simulink model "Sim_Induct_Harmon"  (R2019a)
settings: Solver=FixedStepAuto  StartTime=0.0  StopTime=sim_time  FixedStep=1e-6  MaxStep=1e-4  RelTol=1e-3
values from neighbouring files (symbols this model uses):
  J = 0.0025    [motor_parameters.mat]
  Laq = 0.001    [motor_parameters.mat]
  Lse = 0.001    [motor_parameters.mat]
  Ra = 2.08    [motor_parameters.mat]
  Rse = 5.7    [motor_parameters.mat]
  SEIP4 = [-14.225 -12.275 -10.725 -9.725 -9.1 -8.6 -8.075 -7.65 -7.2 -6.85 -6.492 -6.135 ... (45 elements, 1x45)]    [motor_parameters.mat]
  SEVP4 = [-160 -155 -150 -145 -140 -135 -130 -125 -120 -115 -110 -105 ... (45 elements, 1x45)]    [motor_parameters.mat]
  sim_off = sim_on    [double_load.m]    (also in fourfold_load.m; individual_load.m; triple_load.m)
  sim_on = 50*ones(1,28)    [double_load.m]    (also in fourfold_load.m; individual_load.m; triple_load.m)
  wm0 = 0    [motor_parameters.mat]
  wmo = 157.079632679    [motor_parameters.mat]
undefined symbols (not defined in the file or in its folder): C21, C22, C23, C24, L41, L42, L43, L44, L61, L62, L63, L64, R, R21, R22, R23, R24, R31, R32, R33, R34, R41, R42, R43, R44, R51, R52, R53, R54, R61, R62, R63, R64, R71, R72, R73, R74, Valpha5, Valpha6
libraries: powerlib x225, simulink x72
(part 1 of 3)
settings Model: Creator=USUARIO  LastModifiedBy=USUARIO
settings SolverCC: DecoupledContinuousIntegration=on
settings DataIOCC: ReturnWorkspaceOutputs=off
settings DebuggingCC: ArithmeticOperatorsInVariantConditions=warning
settings SFSimCC: SimUseLocalCustomCode=off
settings RTWCC: RTWUseLocalCustomCode=off

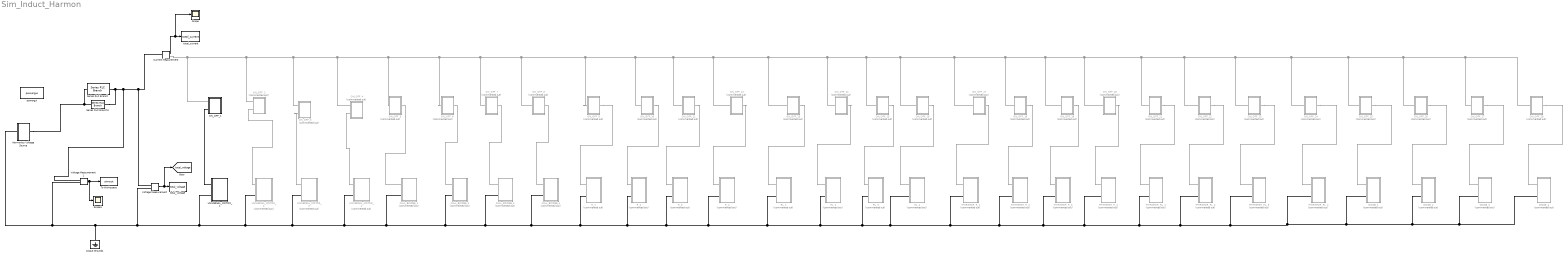
== system Sim_Induct_Harmon ==
  Current Measurement : powerlib/Measurements/Current Measurement  PhasorSimulation=off  OutputType=Complex  PSBequivalent=0
      settings: SourceProductName=Simscape Electrical
  DIODE_1 : Subsystem  Commented=on
  DIODE_2 : Subsystem  Commented=on
  DIODE_3 : Subsystem  Commented=on
  DIODE_4 : Subsystem  Commented=on
  FULL_BRIDGE_1 : Subsystem  Commented=on
  FULL_BRIDGE_2 : Subsystem  Commented=on
  FULL_BRIDGE_3 : Subsystem  Commented=on
  FULL_BRIDGE_4 : Subsystem  Commented=on
  Harmonics Voltage Source : Subsystem
  ON_OFF_1 : Subsystem
  ON_OFF_10 : Subsystem  Commented=on
  ON_OFF_11 : Subsystem  Commented=on
  ON_OFF_12 : Subsystem  Commented=on
  ON_OFF_13 : Subsystem  Commented=on
  ON_OFF_14 : Subsystem  Commented=on
  ON_OFF_15 : Subsystem  Commented=on
  ON_OFF_16 : Subsystem  Commented=on
  ON_OFF_17 : Subsystem  Commented=on
  ON_OFF_18 : Subsystem  Commented=on
  ON_OFF_19 : Subsystem  Commented=on
  ON_OFF_2 : Subsystem  Commented=on
  ON_OFF_20 : Subsystem  Commented=on
  ON_OFF_21 : Subsystem  Commented=on
  ON_OFF_22 : Subsystem  Commented=on
  ON_OFF_23 : Subsystem  Commented=on
  ON_OFF_24 : Subsystem  Commented=on
  ON_OFF_25 : Subsystem  Commented=on
  ON_OFF_26 : Subsystem  Commented=on
  ON_OFF_27 : Subsystem  Commented=on
  ON_OFF_28 : Subsystem  Commented=on
  ON_OFF_3 : Subsystem  Commented=on
  ON_OFF_4 : Subsystem  Commented=on
  ON_OFF_5 : Subsystem  Commented=on
  ON_OFF_6 : Subsystem  Commented=on
  ON_OFF_7 : Subsystem  Commented=on
  ON_OFF_8 : Subsystem  Commented=on
  ON_OFF_9 : Subsystem  Commented=on
  RL_1 : Subsystem  Commented=on
  RL_2 : Subsystem  Commented=on
  RL_3 : Subsystem  Commented=on
  RL_4 : Subsystem  Commented=on
  R_1 : Subsystem  Commented=on
  R_2 : Subsystem  Commented=on
  R_3 : Subsystem  Commented=on
  R_4 : Subsystem  Commented=on
  Scope : Scope
  Scope1 : Scope
  Series RLC Branch : powerlib/Elements/Series RLC Branch  LConnTagsString=__new0  RConnTagsString=__new0  BranchType=RL  Resistance=1e-3  Inductance=1e-3  SetiL0=off  InitialCurrent=0  Capacitance=1e-6  Setx0=off  InitialVoltage=0  Measurements=None
      settings: SourceProductName=Simscape Electrical
  Series RLC Branch1 : powerlib/Elements/Series RLC Branch  LConnTagsString=__new0  RConnTagsString=__new0  BranchType=R  Resistance=3.75e-7  Inductance=1e-12  SetiL0=off  InitialCurrent=0  Capacitance=1e-6  Setx0=off  InitialVoltage=0  Measurements=None
      settings: SourceProductName=Simscape Electrical
  THYRISTOR_RL_1 : Subsystem  Commented=on
  THYRISTOR_RL_2 : Subsystem  Commented=on
  THYRISTOR_RL_3 : Subsystem  Commented=on
  THYRISTOR_RL_4 : Subsystem  Commented=on
  THYRISTOR_R_1 : Subsystem  Commented=on
  THYRISTOR_R_2 : Subsystem  Commented=on
  THYRISTOR_R_3 : Subsystem  Commented=on
  THYRISTOR_R_4 : Subsystem  Commented=on
  To Workspace : ToWorkspace  VariableName=simout  SampleTime=-1
  UNIVERSAL_MOTOR_1 : Subsystem
  UNIVERSAL_MOTOR_2 : Subsystem  Commented=on
  UNIVERSAL_MOTOR_3 : Subsystem  Commented=on
  UNIVERSAL_MOTOR_4 : Subsystem  Commented=on
  Voltage Measurement : powerlib/Measurements/Voltage Measurement  PhasorSimulation=off  OutputType=Complex  PSBequivalent=0
      settings: SourceProductName=Simscape Electrical
  Voltage Measurement1 : powerlib/Measurements/Voltage Measurement  PhasorSimulation=off  OutputType=Complex  PSBequivalent=0
      settings: SourceProductName=Simscape Electrical
  output Ground1 : powerlib/Elements/Ground  LConnTagsString=a
      settings: SourceProductName=Simscape Electrical
  powergui : powerlib/powergui  Priority=1  SimulationMode=Discrete  SampleTime=1e-6  frequency=60  Iterations=100  frequencyindice=0  Pbase=100e6  ErrMax=1e-4  UnitsV=kV  UnitsW=MW  buscounter=0  FunctionMessages=off  echomessages=off  EnableUseOfTLC=off  CurrentSourceSwitches=off  DisableSnubberDevices=off  DisableRonSwitches=off  DisableVfSwitches=off  DisplayEquations=off  AutomaticDiscreteSolvers=off  SolverType=Tustin/Backward Euler (TBE)  Interpol=off  ExternalGateDelay=off  methode=off  Ts=100  x0status=blocks  SPID=off  SwTol=0  HookPort=off  NonlinearTolerance=0  nMaxIteration=15  ContinueOnMaxIteration=off  RestoreLinks=warning  ResistiveCurrentMeasurement=off  Frange=[0:2:500]  Ylog=off  Xlog=on  ShowGrid=off  save=off  variable=ZData  structure=0  ZoomFFT=off  StartTime=0.0  cycles=1  DisplayStyle=1  fundamental=60  FreqAxis=off  MaxFrequency=1000  frequencyindicesteady=1  RmsSteady=1  display=off
      settings: SourceProductName=Simscape Electrical
  total_current : ToWorkspace  VariableName=total_current  SampleTime=-1
  total_voltage : ToWorkspace  VariableName=total_voltage  SampleTime=-1
  tag scope: total_voltage=global
  wires:
  Current Measurement/1 -> Scope/1, total_current/1
  Voltage Measurement/1 -> [total_voltage], total_voltage/1
  Voltage Measurement1/1 -> Scope1/1, To Workspace/1
  connections:
  Harmonics Voltage Source/LConn1 -- Voltage Measurement1/LConn2 -- output Ground1/LConn1 -- Voltage Measurement/LConn2 -- UNIVERSAL_MOTOR_1/LConn2 -- UNIVERSAL_MOTOR_2/LConn2 -- UNIVERSAL_MOTOR_3/LConn2 -- UNIVERSAL_MOTOR_4/LConn2 -- FULL_BRIDGE_4/LConn2 -- R_1/LConn2 -- R_4/LConn2 -- RL_4/LConn2 -- THYRISTOR_R_2/LConn2 -- THYRISTOR_RL_2/LConn2 -- DIODE_3/LConn2 -- DIODE_4/LConn2 -- DIODE_2/LConn2 -- DIODE_1/LConn2 -- THYRISTOR_RL_4/LConn2 -- THYRISTOR_RL_3/LConn2 -- THYRISTOR_RL_1/LConn2 -- THYRISTOR_R_4/LConn2 -- THYRISTOR_R_3/LConn2 -- THYRISTOR_R_1/LConn2 -- RL_3/LConn2 -- RL_2/LConn2 -- RL_1/LConn2 -- R_3/LConn2 -- R_2/LConn2 -- FULL_BRIDGE_3/LConn2 -- FULL_BRIDGE_2/LConn2 -- FULL_BRIDGE_1/LConn2
  Current Measurement/LConn1 -- Voltage Measurement/LConn1 -- Voltage Measurement1/LConn1 -- Series RLC Branch1/RConn1 -- Series RLC Branch/RConn1
  FULL_BRIDGE_1/LConn1 -- ON_OFF_5/RConn1
  ON_OFF_9/RConn1 -- R_1/LConn1
  ON_OFF_13/RConn1 -- RL_1/LConn1
  ON_OFF_17/RConn1 -- THYRISTOR_R_1/LConn1
  ON_OFF_21/RConn1 -- THYRISTOR_RL_1/LConn1
  ON_OFF_14/RConn1 -- RL_2/LConn1
  ON_OFF_15/RConn1 -- RL_3/LConn1
  ON_OFF_16/RConn1 -- RL_4/LConn1
  ON_OFF_18/RConn1 -- THYRISTOR_R_2/LConn1
  ON_OFF_19/RConn1 -- THYRISTOR_R_3/LConn1
  ON_OFF_20/RConn1 -- THYRISTOR_R_4/LConn1
  ON_OFF_22/RConn1 -- THYRISTOR_RL_2/LConn1
  ON_OFF_23/RConn1 -- THYRISTOR_RL_3/LConn1
  ON_OFF_24/RConn1 -- THYRISTOR_RL_4/LConn1
  ON_OFF_10/RConn1 -- R_2/LConn1
  ON_OFF_11/RConn1 -- R_3/LConn1
  ON_OFF_12/RConn1 -- R_4/LConn1
  FULL_BRIDGE_2/LConn1 -- ON_OFF_6/RConn1
  FULL_BRIDGE_3/LConn1 -- ON_OFF_7/RConn1
  FULL_BRIDGE_4/LConn1 -- ON_OFF_8/RConn1
  ON_OFF_25/RConn1 -- DIODE_1/LConn1
  ON_OFF_26/RConn1 -- DIODE_2/LConn1
  ON_OFF_27/RConn1 -- DIODE_3/LConn1
  ON_OFF_28/RConn1 -- DIODE_4/LConn1
  Harmonics Voltage Source/RConn1 -- Series RLC Branch1/LConn1 -- Series RLC Branch/LConn1
  ON_OFF_28/LConn1 -- ON_OFF_27/LConn1 -- ON_OFF_26/LConn1 -- ON_OFF_25/LConn1 -- ON_OFF_24/LConn1 -- ON_OFF_23/LConn1 -- ON_OFF_22/LConn1 -- ON_OFF_21/LConn1 -- ON_OFF_20/LConn1 -- ON_OFF_19/LConn1 -- ON_OFF_18/LConn1 -- ON_OFF_17/LConn1 -- ON_OFF_16/LConn1 -- ON_OFF_15/LConn1 -- ON_OFF_14/LConn1 -- ON_OFF_13/LConn1 -- ON_OFF_12/LConn1 -- ON_OFF_11/LConn1 -- ON_OFF_10/LConn1 -- ON_OFF_9/LConn1 -- ON_OFF_8/LConn1 -- ON_OFF_7/LConn1 -- ON_OFF_6/LConn1 -- Current Measurement/RConn1 -- ON_OFF_1/LConn1 -- ON_OFF_2/LConn1 -- ON_OFF_3/LConn1 -- ON_OFF_4/LConn1 -- ON_OFF_5/LConn1
  ON_OFF_1/LConn2 -- UNIVERSAL_MOTOR_1/LConn1
  ON_OFF_2/LConn2 -- UNIVERSAL_MOTOR_2/LConn1
  ON_OFF_3/LConn2 -- UNIVERSAL_MOTOR_3/LConn1
  ON_OFF_4/LConn2 -- UNIVERSAL_MOTOR_4/LConn1

== system Sim_Induct_Harmon/DIODE_1 ==
  note: LOAD
  Diode : powerlib/Power Electronics/Diode  Ron=0.001  Lon=0  Vf=0.8  IC=0  UseSnubber=0  Rs=500  Cs=250e-9  Measurements=off
      settings: SourceProductName=Simscape Electrical
  Ground2 : powerlib/Elements/Ground  LConnTagsString=a
      settings: SourceProductName=Simscape Electrical
  Scope : Scope
  Scope1 : Scope
  Series RLC Branch : powerlib/Elements/Series RLC Branch  LConnTagsString=__new0  RConnTagsString=__new0  BranchType=R  Resistance=R71  Inductance=1e-3  SetiL0=off  InitialCurrent=0  Capacitance=1e-6  Setx0=off  InitialVoltage=0  Measurements=None
      settings: SourceProductName=Simscape Electrical
  To Workspace1 : ToWorkspace  VariableName=corrente_diodo_1  SampleTime=-1
  To Workspace4 : ToWorkspace  VariableName=tensao_diodo_1  SampleTime=-1
  V_Load : powerlib/Measurements/Voltage Measurement  PhasorSimulation=off  OutputType=Complex  PSBequivalent=0
      settings: SourceProductName=Simscape Electrical
  i_Load : powerlib/Measurements/Current Measurement  Tag=PoWeRsYsTeMmEaSuReMeNt  PhasorSimulation=off  OutputType=Magnitude  PSBequivalent=0
      settings: SourceProductName=Simscape Electrical
  Conn1 : PMIOPort  Side=Left
  Conn2 : PMIOPort  Port=2  Side=Left
  wires:
  i_Load/1 -> To Workspace1/1, Scope1/1
  V_Load/1 -> To Workspace4/1, Scope/1
  connections:
  Series RLC Branch/LConn1 -- Diode/RConn1 -- V_Load/LConn1
  V_Load/LConn2 -- Series RLC Branch/RConn1 -- Conn2/RConn1 -- Ground2/LConn1
  i_Load/RConn1 -- Diode/LConn1
  i_Load/LConn1 -- Conn1/RConn1

== system Sim_Induct_Harmon/DIODE_2 ==
  note: LOAD
  Diode : powerlib/Power Electronics/Diode  Ron=0.001  Lon=0  Vf=0.8  IC=0  UseSnubber=0  Rs=500  Cs=250e-9  Measurements=off
      settings: SourceProductName=Simscape Electrical
  Ground2 : powerlib/Elements/Ground  LConnTagsString=a
      settings: SourceProductName=Simscape Electrical
  Scope : Scope
  Scope1 : Scope
  Series RLC Branch : powerlib/Elements/Series RLC Branch  LConnTagsString=__new0  RConnTagsString=__new0  BranchType=R  Resistance=R72  Inductance=1e-3  SetiL0=off  InitialCurrent=0  Capacitance=1e-6  Setx0=off  InitialVoltage=0  Measurements=None
      settings: SourceProductName=Simscape Electrical
  To Workspace1 : ToWorkspace  VariableName=corrente_diodo_2  SampleTime=-1
  To Workspace4 : ToWorkspace  VariableName=tensao_diodo_2  SampleTime=-1
  V_Load : powerlib/Measurements/Voltage Measurement  PhasorSimulation=off  OutputType=Complex  PSBequivalent=0
      settings: SourceProductName=Simscape Electrical
  i_Load : powerlib/Measurements/Current Measurement  Tag=PoWeRsYsTeMmEaSuReMeNt  PhasorSimulation=off  OutputType=Magnitude  PSBequivalent=0
      settings: SourceProductName=Simscape Electrical
  Conn1 : PMIOPort  Side=Left
  Conn2 : PMIOPort  Port=2  Side=Left
  wires:
  i_Load/1 -> To Workspace1/1, Scope1/1
  V_Load/1 -> To Workspace4/1, Scope/1
  connections:
  Series RLC Branch/LConn1 -- V_Load/LConn1 -- Diode/RConn1
  Series RLC Branch/RConn1 -- V_Load/LConn2 -- Ground2/LConn1 -- Conn2/RConn1
  i_Load/RConn1 -- Diode/LConn1
  i_Load/LConn1 -- Conn1/RConn1

== system Sim_Induct_Harmon/DIODE_3 ==
  note: LOAD
  Diode : powerlib/Power Electronics/Diode  Ron=0.001  Lon=0  Vf=0.8  IC=0  UseSnubber=0  Rs=500  Cs=250e-9  Measurements=off
      settings: SourceProductName=Simscape Electrical
  Ground2 : powerlib/Elements/Ground  LConnTagsString=a
      settings: SourceProductName=Simscape Electrical
  Scope : Scope
  Scope1 : Scope
  Series RLC Branch : powerlib/Elements/Series RLC Branch  LConnTagsString=__new0  RConnTagsString=__new0  BranchType=R  Resistance=R73  Inductance=1e-3  SetiL0=off  InitialCurrent=0  Capacitance=1e-6  Setx0=off  InitialVoltage=0  Measurements=None
      settings: SourceProductName=Simscape Electrical
  To Workspace1 : ToWorkspace  VariableName=corrente_diodo_3  SampleTime=-1
  To Workspace4 : ToWorkspace  VariableName=tensao_diodo_3  SampleTime=-1
  V_Load : powerlib/Measurements/Voltage Measurement  PhasorSimulation=off  OutputType=Complex  PSBequivalent=0
      settings: SourceProductName=Simscape Electrical
  i_Load : powerlib/Measurements/Current Measurement  Tag=PoWeRsYsTeMmEaSuReMeNt  PhasorSimulation=off  OutputType=Magnitude  PSBequivalent=0
      settings: SourceProductName=Simscape Electrical
  Conn1 : PMIOPort  Side=Left
  Conn2 : PMIOPort  Port=2  Side=Left
  wires:
  i_Load/1 -> To Workspace1/1, Scope1/1
  V_Load/1 -> To Workspace4/1, Scope/1
  connections:
  Series RLC Branch/LConn1 -- V_Load/LConn1 -- Diode/RConn1
  Series RLC Branch/RConn1 -- V_Load/LConn2 -- Ground2/LConn1 -- Conn2/RConn1
  i_Load/RConn1 -- Diode/LConn1
  i_Load/LConn1 -- Conn1/RConn1

== system Sim_Induct_Harmon/DIODE_4 ==
  note: LOAD
  Diode : powerlib/Power Electronics/Diode  Ron=0.001  Lon=0  Vf=0.8  IC=0  UseSnubber=0  Rs=500  Cs=250e-9  Measurements=off
      settings: SourceProductName=Simscape Electrical
  Ground2 : powerlib/Elements/Ground  LConnTagsString=a
      settings: SourceProductName=Simscape Electrical
  Scope : Scope
  Scope1 : Scope
  Series RLC Branch : powerlib/Elements/Series RLC Branch  LConnTagsString=__new0  RConnTagsString=__new0  BranchType=R  Resistance=R74  Inductance=1e-3  SetiL0=off  InitialCurrent=0  Capacitance=1e-6  Setx0=off  InitialVoltage=0  Measurements=None
      settings: SourceProductName=Simscape Electrical
  To Workspace1 : ToWorkspace  VariableName=corrente_diodo_4  SampleTime=-1
  To Workspace4 : ToWorkspace  VariableName=tensao_diodo_4  SampleTime=-1
  V_Load : powerlib/Measurements/Voltage Measurement  PhasorSimulation=off  OutputType=Complex  PSBequivalent=0
      settings: SourceProductName=Simscape Electrical
  i_Load : powerlib/Measurements/Current Measurement  Tag=PoWeRsYsTeMmEaSuReMeNt  PhasorSimulation=off  OutputType=Magnitude  PSBequivalent=0
      settings: SourceProductName=Simscape Electrical
  Conn1 : PMIOPort  Side=Left
  Conn2 : PMIOPort  Port=2  Side=Left
  wires:
  i_Load/1 -> To Workspace1/1, Scope1/1
  V_Load/1 -> To Workspace4/1, Scope/1
  connections:
  Series RLC Branch/LConn1 -- V_Load/LConn1 -- Diode/RConn1
  Series RLC Branch/RConn1 -- V_Load/LConn2 -- Ground2/LConn1 -- Conn2/RConn1
  i_Load/RConn1 -- Diode/LConn1
  i_Load/LConn1 -- Conn1/RConn1

== system Sim_Induct_Harmon/FULL_BRIDGE_1 ==
  Diode{,1..3} (4 alike) : powerlib/Power Electronics/Diode  Ron=0.001  Lon=0  Vf=0.8  IC=0  UseSnubber=0  Rs=500  Cs=250e-9  Measurements=off
      settings: SourceProductName=Simscape Electrical
  Scope : Scope
  Scope1 : Scope
  Series RLC Branch : powerlib/Elements/Series RLC Branch  LConnTagsString=__new0  RConnTagsString=__new0  BranchType=C  Resistance=R  Inductance=1e-3  SetiL0=off  InitialCurrent=0  Capacitance=C21  Setx0=off  InitialVoltage=0  Measurements=None
      settings: SourceProductName=Simscape Electrical
  Series RLC Branch1 : powerlib/Elements/Series RLC Branch  LConnTagsString=__new0  RConnTagsString=__new0  BranchType=R  Resistance=R21  Inductance=1e-3  SetiL0=off  InitialCurrent=0  Capacitance=1e-6  Setx0=off  InitialVoltage=0  Measurements=None
      settings: SourceProductName=Simscape Electrical
  Series RLC Branch2 : powerlib/Elements/Series RLC Branch  LConnTagsString=__new0  RConnTagsString=__new0  BranchType=R  Resistance=10  Inductance=1e-3  SetiL0=off  InitialCurrent=0  Capacitance=C21  Setx0=off  InitialVoltage=0  Measurements=None
      settings: SourceProductName=Simscape Electrical
  To Workspace1 : ToWorkspace  VariableName=corrente_ponte_1  SampleTime=-1
  To Workspace4 : ToWorkspace  VariableName=tensao_ponte_1  SampleTime=-1
  V_Load : powerlib/Measurements/Voltage Measurement  PhasorSimulation=off  OutputType=Complex  PSBequivalent=0
      settings: SourceProductName=Simscape Electrical
  i_Load : powerlib/Measurements/Current Measurement  Tag=PoWeRsYsTeMmEaSuReMeNt  PhasorSimulation=off  OutputType=Magnitude  PSBequivalent=0
      settings: SourceProductName=Simscape Electrical
  Conn1 : PMIOPort  Side=Left
  Conn2 : PMIOPort  Port=2  Side=Left
  wires:
  i_Load/1 -> To Workspace1/1, Scope1/1
  V_Load/1 -> To Workspace4/1, Scope/1
  connections:
  Conn1/RConn1 -- i_Load/LConn1
  Diode1/LConn1 -- Conn2/RConn1 -- Diode3/RConn1
  Series RLC Branch/LConn1 -- Diode/RConn1 -- Diode1/RConn1 -- V_Load/LConn1 -- Series RLC Branch1/LConn1
  Series RLC Branch/RConn1 -- Diode2/LConn1 -- Diode3/LConn1 -- V_Load/LConn2 -- Series RLC Branch1/RConn1
  Series RLC Branch2/RConn1 -- Diode2/RConn1 -- Diode/LConn1
  i_Load/RConn1 -- Series RLC Branch2/LConn1

== system Sim_Induct_Harmon/FULL_BRIDGE_2 ==
  Diode{,1..3} (4 alike) : powerlib/Power Electronics/Diode  Ron=0.001  Lon=0  Vf=0.8  IC=0  UseSnubber=0  Rs=500  Cs=250e-9  Measurements=off
      settings: SourceProductName=Simscape Electrical
  Scope : Scope
  Scope1 : Scope
  Series RLC Branch : powerlib/Elements/Series RLC Branch  LConnTagsString=__new0  RConnTagsString=__new0  BranchType=C  Resistance=R  Inductance=1e-3  SetiL0=off  InitialCurrent=0  Capacitance=C22  Setx0=off  InitialVoltage=0  Measurements=None
      settings: SourceProductName=Simscape Electrical
  Series RLC Branch1 : powerlib/Elements/Series RLC Branch  LConnTagsString=__new0  RConnTagsString=__new0  BranchType=R  Resistance=R22  Inductance=1e-3  SetiL0=off  InitialCurrent=0  Capacitance=1e-6  Setx0=off  InitialVoltage=0  Measurements=None
      settings: SourceProductName=Simscape Electrical
  Series RLC Branch2 : powerlib/Elements/Series RLC Branch  LConnTagsString=__new0  RConnTagsString=__new0  BranchType=R  Resistance=10  Inductance=1e-3  SetiL0=off  InitialCurrent=0  Capacitance=C21  Setx0=off  InitialVoltage=0  Measurements=None
      settings: SourceProductName=Simscape Electrical
  To Workspace1 : ToWorkspace  VariableName=corrente_ponte_2  SampleTime=-1
  To Workspace4 : ToWorkspace  VariableName=tensao_ponte_2  SampleTime=-1
  V_Load : powerlib/Measurements/Voltage Measurement  PhasorSimulation=off  OutputType=Complex  PSBequivalent=0
      settings: SourceProductName=Simscape Electrical
  i_Load : powerlib/Measurements/Current Measurement  Tag=PoWeRsYsTeMmEaSuReMeNt  PhasorSimulation=off  OutputType=Magnitude  PSBequivalent=0
      settings: SourceProductName=Simscape Electrical
  Conn1 : PMIOPort  Side=Left
  Conn2 : PMIOPort  Port=2  Side=Left
  wires:
  i_Load/1 -> To Workspace1/1, Scope1/1
  V_Load/1 -> To Workspace4/1, Scope/1
  connections:
  Conn1/RConn1 -- i_Load/LConn1
  Diode1/LConn1 -- Conn2/RConn1 -- Diode3/RConn1
  Series RLC Branch/LConn1 -- Diode/RConn1 -- Diode1/RConn1 -- V_Load/LConn1 -- Series RLC Branch1/LConn1
  Series RLC Branch/RConn1 -- Diode2/LConn1 -- Diode3/LConn1 -- V_Load/LConn2 -- Series RLC Branch1/RConn1
  Diode2/RConn1 -- Series RLC Branch2/RConn1 -- Diode/LConn1
  i_Load/RConn1 -- Series RLC Branch2/LConn1

== system Sim_Induct_Harmon/FULL_BRIDGE_3 ==
  Diode{,1..3} (4 alike) : powerlib/Power Electronics/Diode  Ron=0.001  Lon=0  Vf=0.8  IC=0  UseSnubber=0  Rs=500  Cs=250e-9  Measurements=off
      settings: SourceProductName=Simscape Electrical
  Scope : Scope
  Scope1 : Scope
  Series RLC Branch : powerlib/Elements/Series RLC Branch  LConnTagsString=__new0  RConnTagsString=__new0  BranchType=C  Resistance=R  Inductance=1e-3  SetiL0=off  InitialCurrent=0  Capacitance=C23  Setx0=off  InitialVoltage=0  Measurements=None
      settings: SourceProductName=Simscape Electrical
  Series RLC Branch1 : powerlib/Elements/Series RLC Branch  LConnTagsString=__new0  RConnTagsString=__new0  BranchType=R  Resistance=R23  Inductance=1e-3  SetiL0=off  InitialCurrent=0  Capacitance=1e-6  Setx0=off  InitialVoltage=0  Measurements=None
      settings: SourceProductName=Simscape Electrical
  Series RLC Branch2 : powerlib/Elements/Series RLC Branch  LConnTagsString=__new0  RConnTagsString=__new0  BranchType=R  Resistance=10  Inductance=1e-3  SetiL0=off  InitialCurrent=0  Capacitance=C21  Setx0=off  InitialVoltage=0  Measurements=None
      settings: SourceProductName=Simscape Electrical
  To Workspace1 : ToWorkspace  VariableName=corrente_ponte_3  SampleTime=-1
  To Workspace4 : ToWorkspace  VariableName=tensao_ponte_3  SampleTime=-1
  V_Load : powerlib/Measurements/Voltage Measurement  PhasorSimulation=off  OutputType=Complex  PSBequivalent=0
      settings: SourceProductName=Simscape Electrical
  i_Load : powerlib/Measurements/Current Measurement  Tag=PoWeRsYsTeMmEaSuReMeNt  PhasorSimulation=off  OutputType=Magnitude  PSBequivalent=0
      settings: SourceProductName=Simscape Electrical
  powergui : powerlib/powergui  Priority=1  SimulationMode=Discrete  SampleTime=1e-6  frequency=60  Iterations=100  frequencyindice=60  Pbase=100e6  ErrMax=1e-4  UnitsV=kV  UnitsW=MW  buscounter=0  FunctionMessages=off  echomessages=off  EnableUseOfTLC=off  CurrentSourceSwitches=off  DisableSnubberDevices=off  DisableRonSwitches=off  DisableVfSwitches=off  DisplayEquations=off  SolverType=Tustin/Backward Euler (TBE)  Interpol=off  ExternalGateDelay=off  methode=off  Ts=100  x0status=zero  SPID=off  SwTol=0  HookPort=off  RestoreLinks=warning  ResistiveCurrentMeasurement=off  Frange=[0:2:500]  Ylog=off  Xlog=on  ShowGrid=off  save=off  variable=ZData  structure=0  ZoomFFT=off  StartTime=0.0  cycles=1  DisplayStyle=1  fundamental=60  FreqAxis=off  MaxFrequency=1000  frequencyindicesteady=1  RmsSteady=1  display=off
      settings: SourceProductName=Simscape Electrical
  Conn1 : PMIOPort  Side=Left
  Conn2 : PMIOPort  Port=2  Side=Left
  wires:
  i_Load/1 -> To Workspace1/1, Scope1/1
  V_Load/1 -> To Workspace4/1, Scope/1
  connections:
  Conn1/RConn1 -- i_Load/LConn1
  Diode1/LConn1 -- Conn2/RConn1 -- Diode3/RConn1
  Series RLC Branch/LConn1 -- Diode/RConn1 -- Diode1/RConn1 -- V_Load/LConn1 -- Series RLC Branch1/LConn1
  Series RLC Branch/RConn1 -- Diode2/LConn1 -- Diode3/LConn1 -- V_Load/LConn2 -- Series RLC Branch1/RConn1
  Diode/LConn1 -- Series RLC Branch2/RConn1 -- Diode2/RConn1
  i_Load/RConn1 -- Series RLC Branch2/LConn1

== system Sim_Induct_Harmon/FULL_BRIDGE_4 ==
  Diode{,1..3} (4 alike) : powerlib/Power Electronics/Diode  Ron=0.001  Lon=0  Vf=0.8  IC=0  UseSnubber=0  Rs=500  Cs=250e-9  Measurements=off
      settings: SourceProductName=Simscape Electrical
  Scope : Scope
  Scope1 : Scope
  Series RLC Branch : powerlib/Elements/Series RLC Branch  LConnTagsString=__new0  RConnTagsString=__new0  BranchType=C  Resistance=R  Inductance=1e-3  SetiL0=off  InitialCurrent=0  Capacitance=C24  Setx0=off  InitialVoltage=0  Measurements=None
      settings: SourceProductName=Simscape Electrical
  Series RLC Branch1 : powerlib/Elements/Series RLC Branch  LConnTagsString=__new0  RConnTagsString=__new0  BranchType=R  Resistance=R24  Inductance=1e-3  SetiL0=off  InitialCurrent=0  Capacitance=1e-6  Setx0=off  InitialVoltage=0  Measurements=None
      settings: SourceProductName=Simscape Electrical
  Series RLC Branch2 : powerlib/Elements/Series RLC Branch  LConnTagsString=__new0  RConnTagsString=__new0  BranchType=R  Resistance=10  Inductance=1e-3  SetiL0=off  InitialCurrent=0  Capacitance=C21  Setx0=off  InitialVoltage=0  Measurements=None
      settings: SourceProductName=Simscape Electrical
  To Workspace1 : ToWorkspace  VariableName=corrente_ponte_4  SampleTime=-1
  To Workspace4 : ToWorkspace  VariableName=tensao_ponte_4  SampleTime=-1
  V_Load : powerlib/Measurements/Voltage Measurement  PhasorSimulation=off  OutputType=Complex  PSBequivalent=0
      settings: SourceProductName=Simscape Electrical
  i_Load : powerlib/Measurements/Current Measurement  Tag=PoWeRsYsTeMmEaSuReMeNt  PhasorSimulation=off  OutputType=Magnitude  PSBequivalent=0
      settings: SourceProductName=Simscape Electrical
  Conn1 : PMIOPort  Side=Left
  Conn2 : PMIOPort  Port=2  Side=Left
  wires:
  i_Load/1 -> To Workspace1/1, Scope1/1
  V_Load/1 -> To Workspace4/1, Scope/1
  connections:
  Conn1/RConn1 -- i_Load/LConn1
  Diode1/LConn1 -- Conn2/RConn1 -- Diode3/RConn1
  Series RLC Branch/LConn1 -- Diode/RConn1 -- Diode1/RConn1 -- V_Load/LConn1 -- Series RLC Branch1/LConn1
  Series RLC Branch/RConn1 -- Diode2/LConn1 -- Diode3/LConn1 -- V_Load/LConn2 -- Series RLC Branch1/RConn1
  Diode/LConn1 -- Series RLC Branch2/RConn1 -- Diode2/RConn1
  i_Load/RConn1 -- Series RLC Branch2/LConn1

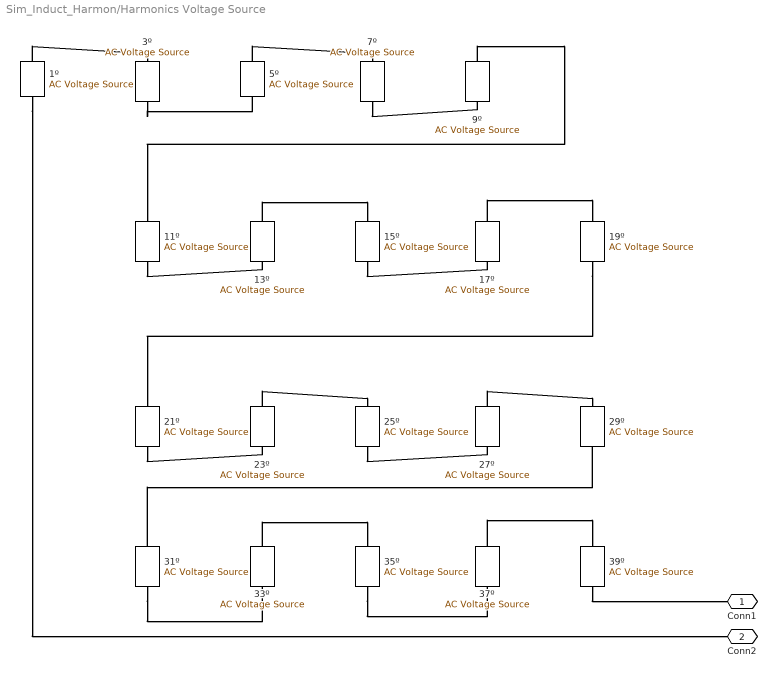
== system Sim_Induct_Harmon/Harmonics Voltage Source ==
  11º : powerlib/Electrical Sources/AC Voltage Source  Amplitude=0.242776489233398  Phase=-58.1113  Frequency=660  SampleTime=0  Measurements=None  BusType=swing  Pref=10e3  Qref=0  Qmin=-inf  Qmax=+inf
      settings: SourceProductName=Simscape Electrical
  13º : powerlib/Electrical Sources/AC Voltage Source  Amplitude=0.492098307543115  Phase=-106.3644  Frequency=780  SampleTime=0  Measurements=None  BusType=swing  Pref=10e3  Qref=0  Qmin=-inf  Qmax=+inf
      settings: SourceProductName=Simscape Electrical
  15º : powerlib/Electrical Sources/AC Voltage Source  Amplitude=0.778923261571752  Phase=75.8084  Frequency=900  SampleTime=0  Measurements=None  BusType=swing  Pref=10e3  Qref=0  Qmin=-inf  Qmax=+inf
      settings: SourceProductName=Simscape Electrical
  17º : powerlib/Electrical Sources/AC Voltage Source  Amplitude=0.160351450954246  Phase=-10.1854  Frequency=1020  SampleTime=0  Measurements=None  BusType=swing  Pref=10e3  Qref=0  Qmin=-inf  Qmax=+inf
      settings: SourceProductName=Simscape Electrical
  19º : powerlib/Electrical Sources/AC Voltage Source  Amplitude=0.0278424562249700  Phase=126.3291  Frequency=1140  SampleTime=0  Measurements=None  BusType=swing  Pref=10e3  Qref=0  Qmin=-inf  Qmax=+inf
      settings: SourceProductName=Simscape Electrical
  1º : powerlib/Electrical Sources/AC Voltage Source  Amplitude=179  Phase=-30.1588  Frequency=60  SampleTime=0  Measurements=None  BusType=swing  Pref=10e3  Qref=0  Qmin=-inf  Qmax=+inf
      settings: SourceProductName=Simscape Electrical
  21º : powerlib/Electrical Sources/AC Voltage Source  Amplitude=0.222530962077158  Phase=-79.4995  Frequency=1260  SampleTime=0  Measurements=None  BusType=swing  Pref=10e3  Qref=0  Qmin=-inf  Qmax=+inf
      settings: SourceProductName=Simscape Electrical
  23º : powerlib/Electrical Sources/AC Voltage Source  Amplitude=0.0418274495996007  Phase=86.3490  Frequency=1380  SampleTime=0  Measurements=None  BusType=swing  Pref=10e3  Qref=0  Qmin=-inf  Qmax=+inf
      settings: SourceProductName=Simscape Electrical
  25º : powerlib/Electrical Sources/AC Voltage Source  Amplitude=0.110851490163759  Phase=57.6427  Frequency=1500  SampleTime=0  Measurements=None  BusType=swing  Pref=10e3  Qref=0  Qmin=-inf  Qmax=+inf
      settings: SourceProductName=Simscape Electrical
  27º : powerlib/Electrical Sources/AC Voltage Source  Amplitude=0.0778617078813013  Phase=173.5639  Frequency=1620  SampleTime=0  Measurements=None  BusType=swing  Pref=10e3  Qref=0  Qmin=-inf  Qmax=+inf
      settings: SourceProductName=Simscape Electrical
  29º : powerlib/Electrical Sources/AC Voltage Source  Amplitude=0.0894234496049604  Phase=148.6408  Frequency=1740  SampleTime=0  Measurements=None  BusType=swing  Pref=10e3  Qref=0  Qmin=-inf  Qmax=+inf
      settings: SourceProductName=Simscape Electrical
  31º : powerlib/Electrical Sources/AC Voltage Source  Amplitude=0.0975741619325717  Phase=-92.8788  Frequency=1860  SampleTime=0  Measurements=None  BusType=swing  Pref=10e3  Qref=0  Qmin=-inf  Qmax=+inf
      settings: SourceProductName=Simscape Electrical
  33º : powerlib/Electrical Sources/AC Voltage Source  Amplitude=0.0150692109662702  Phase=38.3346  Frequency=1980  SampleTime=0  Measurements=None  BusType=swing  Pref=10e3  Qref=0  Qmin=-inf  Qmax=+inf
      settings: SourceProductName=Simscape Electrical
  35º : powerlib/Electrical Sources/AC Voltage Source  Amplitude=0.0548604672040831  Phase=16.6025  Frequency=2100  SampleTime=0  Measurements=None  BusType=swing  Pref=10e3  Qref=0  Qmin=-inf  Qmax=+inf
      settings: SourceProductName=Simscape Electrical
  37º : powerlib/Electrical Sources/AC Voltage Source  Amplitude=0.0505087506298168  Phase=87.0202  Frequency=2220  SampleTime=0  Measurements=None  BusType=swing  Pref=10e3  Qref=0  Qmin=-inf  Qmax=+inf
      settings: SourceProductName=Simscape Electrical
  39º : powerlib/Electrical Sources/AC Voltage Source  Amplitude=0.0425905748970170  Phase=90.8832  Frequency=2340  SampleTime=0  Measurements=None  BusType=swing  Pref=10e3  Qref=0  Qmin=-inf  Qmax=+inf
      settings: SourceProductName=Simscape Electrical
  3º : powerlib/Electrical Sources/AC Voltage Source  Amplitude=3.58785003983961  Phase=17.6777  Frequency=180  SampleTime=0  Measurements=None  BusType=swing  Pref=10e3  Qref=0  Qmin=-inf  Qmax=+inf
      settings: SourceProductName=Simscape Electrical
  5º : powerlib/Electrical Sources/AC Voltage Source  Amplitude=4.50339362685229  Phase=22.7344  Frequency=300  SampleTime=0  Measurements=None  BusType=swing  Pref=10e3  Qref=0  Qmin=-inf  Qmax=+inf
      settings: SourceProductName=Simscape Electrical
  7º : powerlib/Electrical Sources/AC Voltage Source  Amplitude=1.04825083702916  Phase=179.6309  Frequency=420  SampleTime=0  Measurements=None  BusType=swing  Pref=10e3  Qref=0  Qmin=-inf  Qmax=+inf
      settings: SourceProductName=Simscape Electrical
  9º : powerlib/Electrical Sources/AC Voltage Source  Amplitude=2.09509433966437  Phase=-143.5761  Frequency=540  SampleTime=0  Measurements=None  BusType=swing  Pref=10e3  Qref=0  Qmin=-inf  Qmax=+inf
      settings: SourceProductName=Simscape Electrical
  Conn1 : PMIOPort  Side=Right
  Conn2 : PMIOPort  Port=2  Side=Left
  connections:
  1º/LConn1 -- Conn2/RConn1
  1º/RConn1 -- 3º/LConn1
  3º/RConn1 -- 5º/LConn1
  5º/RConn1 -- 7º/LConn1
  7º/RConn1 -- 9º/LConn1
  9º/RConn1 -- 11º/LConn1
  11º/RConn1 -- 13º/LConn1
  13º/RConn1 -- 15º/LConn1
  15º/RConn1 -- 17º/LConn1
  17º/RConn1 -- 19º/LConn1
  19º/RConn1 -- 21º/LConn1
  21º/RConn1 -- 23º/LConn1
  23º/RConn1 -- 25º/LConn1
  25º/RConn1 -- 27º/LConn1
  27º/RConn1 -- 29º/LConn1
  31º/LConn1 -- 29º/RConn1
  31º/RConn1 -- 33º/LConn1
  33º/RConn1 -- 35º/LConn1
  35º/RConn1 -- 37º/LConn1
  37º/RConn1 -- 39º/LConn1
  39º/RConn1 -- Conn1/RConn1

== system Sim_Induct_Harmon/ON_OFF_1 ==
  Clock1 : Clock
  Clock2 : Clock
  Clock3 : Clock
  Compare To Constant : simulink/Logic and Bit Operations/Compare To Constant  relop=>=  const=sim_on(1)  OutDataTypeStr=boolean
  Compare To Constant1 : simulink/Logic and Bit Operations/Compare To Constant  relop=>=  const=sim_off(1)  OutDataTypeStr=boolean
  Compare To Constant2 : simulink/Logic and Bit Operations/Compare To Constant  relop=>=  const=sim_on(1)  OutDataTypeStr=boolean
  Constant : Constant  Value=0
  Constant1 : Constant  Value=0
  Ideal Switch : powerlib/Power Electronics/Ideal Switch  Ron=0.001  Lon=0  IC=0  Rs=1e5  Cs=inf  Measurements=off
      settings: SourceProductName=Simscape Electrical
  Series RLC Branch : powerlib/Elements/Series RLC Branch  LConnTagsString=__new0  RConnTagsString=__new0  BranchType=R  Resistance=1e-10  Inductance=1e-3  SetiL0=off  InitialCurrent=0  Capacitance=1e-6  Setx0=off  InitialVoltage=0  Measurements=None
      settings: SourceProductName=Simscape Electrical
  Switch : Switch
  Switch1 : Switch
  Conn1 : PMIOPort  Side=Left
  Conn2 : PMIOPort  Port=2  Side=Left
  tag scope: tensao_1=global
  wires:
  Switch1/1 -> [tensao_1]
  Constant/1 -> Switch/3
  Switch/1 -> Switch1/3
  Clock1/1 -> Compare To Constant/1
  Clock2/1 -> Compare To Constant1/1
  Compare To Constant1/1 -> Switch1/2
  [fonte_tensao] -> Switch/1
  Constant1/1 -> Switch1/1
  Compare To Constant/1 -> Switch/2
  Clock3/1 -> Compare To Constant2/1
  Compare To Constant2/1 -> Ideal Switch/1
  connections:
  Conn1/RConn1 -- Ideal Switch/LConn1
  Series RLC Branch/RConn1 -- Conn2/RConn1
  Ideal Switch/RConn1 -- Series RLC Branch/LConn1

== system Sim_Induct_Harmon/ON_OFF_10 ==
  Clock4 : Clock
  Compare To Constant2 : simulink/Logic and Bit Operations/Compare To Constant  relop=>=  const=sim_on(10)  OutDataTypeStr=boolean
  Compare To Constat3 : simulink/Logic and Bit Operations/Compare To Constant  relop=<=  const=sim_off(10)  OutDataTypeStr=boolean
  OFF2 : powerlib/Power Electronics/Ideal Switch  Ron=0.001  Lon=0  IC=0  Rs=1e5  Cs=inf  Measurements=off
      settings: SourceProductName=Simscape Electrical
  ON2 : powerlib/Power Electronics/Ideal Switch  Ron=0.001  Lon=0  IC=0  Rs=1e5  Cs=inf  Measurements=off
      settings: SourceProductName=Simscape Electrical
  Conn1 : PMIOPort  Side=Left
  Conn2 : PMIOPort  Port=2  Side=Right
  wires:
  Compare To Constant2/1 -> ON2/1
  Compare To Constat3/1 -> OFF2/1
  Clock4/1 -> Compare To Constat3/1, Compare To Constant2/1
  connections:
  OFF2/RConn1 -- Conn2/RConn1
  ON2/RConn1 -- OFF2/LConn1
  ON2/LConn1 -- Conn1/RConn1

== system Sim_Induct_Harmon/ON_OFF_11 ==
  Clock4 : Clock
  Compare To Constant2 : simulink/Logic and Bit Operations/Compare To Constant  relop=>=  const=sim_on(11)  OutDataTypeStr=boolean
  Compare To Constat3 : simulink/Logic and Bit Operations/Compare To Constant  relop=<=  const=sim_off(11)  OutDataTypeStr=boolean
  OFF2 : powerlib/Power Electronics/Ideal Switch  Ron=0.001  Lon=0  IC=0  Rs=1e5  Cs=inf  Measurements=off
      settings: SourceProductName=Simscape Electrical
  ON2 : powerlib/Power Electronics/Ideal Switch  Ron=0.001  Lon=0  IC=0  Rs=1e5  Cs=inf  Measurements=off
      settings: SourceProductName=Simscape Electrical
  Conn1 : PMIOPort  Side=Left
  Conn2 : PMIOPort  Port=2  Side=Right
  wires:
  Compare To Constant2/1 -> ON2/1
  Compare To Constat3/1 -> OFF2/1
  Clock4/1 -> Compare To Constat3/1, Compare To Constant2/1
  connections:
  OFF2/RConn1 -- Conn2/RConn1
  ON2/RConn1 -- OFF2/LConn1
  ON2/LConn1 -- Conn1/RConn1

== system Sim_Induct_Harmon/ON_OFF_12 ==
  Clock4 : Clock
  Compare To Constant2 : simulink/Logic and Bit Operations/Compare To Constant  relop=>=  const=sim_on(12)  OutDataTypeStr=boolean
  Compare To Constat3 : simulink/Logic and Bit Operations/Compare To Constant  relop=<=  const=sim_off(12)  OutDataTypeStr=boolean
  OFF2 : powerlib/Power Electronics/Ideal Switch  Ron=0.001  Lon=0  IC=0  Rs=1e5  Cs=inf  Measurements=off
      settings: SourceProductName=Simscape Electrical
  ON2 : powerlib/Power Electronics/Ideal Switch  Ron=0.001  Lon=0  IC=0  Rs=1e5  Cs=inf  Measurements=off
      settings: SourceProductName=Simscape Electrical
  Conn1 : PMIOPort  Side=Left
  Conn2 : PMIOPort  Port=2  Side=Right
  wires:
  Compare To Constant2/1 -> ON2/1
  Compare To Constat3/1 -> OFF2/1
  Clock4/1 -> Compare To Constat3/1, Compare To Constant2/1
  connections:
  OFF2/RConn1 -- Conn2/RConn1
  ON2/RConn1 -- OFF2/LConn1
  ON2/LConn1 -- Conn1/RConn1

== system Sim_Induct_Harmon/ON_OFF_13 ==
  Clock6 : Clock
  Compare To Constant3 : simulink/Logic and Bit Operations/Compare To Constant  relop=>=  const=sim_on(13)  OutDataTypeStr=boolean
  Compare To Constat4 : simulink/Logic and Bit Operations/Compare To Constant  relop=<=  const=sim_off(13)  OutDataTypeStr=boolean
  OFF3 : powerlib/Power Electronics/Ideal Switch  Ron=0.001  Lon=0  IC=0  Rs=1e5  Cs=inf  Measurements=off
      settings: SourceProductName=Simscape Electrical
  ON3 : powerlib/Power Electronics/Ideal Switch  Ron=0.001  Lon=0  IC=0  Rs=1e5  Cs=inf  Measurements=off
      settings: SourceProductName=Simscape Electrical
  Conn1 : PMIOPort  Side=Left
  Conn2 : PMIOPort  Port=2  Side=Right
  wires:
  Compare To Constant3/1 -> ON3/1
  Clock6/1 -> Compare To Constat4/1, Compare To Constant3/1
  Compare To Constat4/1 -> OFF3/1
  connections:
  ON3/RConn1 -- OFF3/LConn1
  OFF3/RConn1 -- Conn2/RConn1
  ON3/LConn1 -- Conn1/RConn1

== system Sim_Induct_Harmon/ON_OFF_14 ==
  Clock6 : Clock
  Compare To Constant3 : simulink/Logic and Bit Operations/Compare To Constant  relop=>=  const=sim_on(14)  OutDataTypeStr=boolean
  Compare To Constat4 : simulink/Logic and Bit Operations/Compare To Constant  relop=<=  const=sim_off(14)  OutDataTypeStr=boolean
  OFF3 : powerlib/Power Electronics/Ideal Switch  Ron=0.001  Lon=0  IC=0  Rs=1e5  Cs=inf  Measurements=off
      settings: SourceProductName=Simscape Electrical
  ON3 : powerlib/Power Electronics/Ideal Switch  Ron=0.001  Lon=0  IC=0  Rs=1e5  Cs=inf  Measurements=off
      settings: SourceProductName=Simscape Electrical
  Conn1 : PMIOPort  Side=Left
  Conn2 : PMIOPort  Port=2  Side=Right
  wires:
  Compare To Constant3/1 -> ON3/1
  Clock6/1 -> Compare To Constat4/1, Compare To Constant3/1
  Compare To Constat4/1 -> OFF3/1
  connections:
  ON3/RConn1 -- OFF3/LConn1
  OFF3/RConn1 -- Conn2/RConn1
  ON3/LConn1 -- Conn1/RConn1

== system Sim_Induct_Harmon/ON_OFF_15 ==
  Clock6 : Clock
  Compare To Constant3 : simulink/Logic and Bit Operations/Compare To Constant  relop=>=  const=sim_on(15)  OutDataTypeStr=boolean
  Compare To Constat4 : simulink/Logic and Bit Operations/Compare To Constant  relop=<=  const=sim_off(15)  OutDataTypeStr=boolean
  OFF3 : powerlib/Power Electronics/Ideal Switch  Ron=0.001  Lon=0  IC=0  Rs=1e5  Cs=inf  Measurements=off
      settings: SourceProductName=Simscape Electrical
  ON3 : powerlib/Power Electronics/Ideal Switch  Ron=0.001  Lon=0  IC=0  Rs=1e5  Cs=inf  Measurements=off
      settings: SourceProductName=Simscape Electrical
  Conn1 : PMIOPort  Side=Left
  Conn2 : PMIOPort  Port=2  Side=Right
  wires:
  Compare To Constant3/1 -> ON3/1
  Clock6/1 -> Compare To Constat4/1, Compare To Constant3/1
  Compare To Constat4/1 -> OFF3/1
  connections:
  ON3/RConn1 -- OFF3/LConn1
  OFF3/RConn1 -- Conn2/RConn1
  ON3/LConn1 -- Conn1/RConn1

== system Sim_Induct_Harmon/ON_OFF_16 ==
  Clock6 : Clock
  Compare To Constant3 : simulink/Logic and Bit Operations/Compare To Constant  relop=>=  const=sim_on(16)  OutDataTypeStr=boolean
  Compare To Constat4 : simulink/Logic and Bit Operations/Compare To Constant  relop=<=  const=sim_off(16)  OutDataTypeStr=boolean
  OFF3 : powerlib/Power Electronics/Ideal Switch  Ron=0.001  Lon=0  IC=0  Rs=1e5  Cs=inf  Measurements=off
      settings: SourceProductName=Simscape Electrical
  ON3 : powerlib/Power Electronics/Ideal Switch  Ron=0.001  Lon=0  IC=0  Rs=1e5  Cs=inf  Measurements=off
      settings: SourceProductName=Simscape Electrical
  Conn1 : PMIOPort  Side=Left
  Conn2 : PMIOPort  Port=2  Side=Right
  wires:
  Compare To Constant3/1 -> ON3/1
  Clock6/1 -> Compare To Constat4/1, Compare To Constant3/1
  Compare To Constat4/1 -> OFF3/1
  connections:
  ON3/RConn1 -- OFF3/LConn1
  OFF3/RConn1 -- Conn2/RConn1
  ON3/LConn1 -- Conn1/RConn1

== system Sim_Induct_Harmon/ON_OFF_17 ==
  Clock7 : Clock
  Compare To Constant4 : simulink/Logic and Bit Operations/Compare To Constant  relop=>=  const=sim_on(17)  OutDataTypeStr=boolean
  Compare To Constat5 : simulink/Logic and Bit Operations/Compare To Constant  relop=<=  const=sim_off(17)  OutDataTypeStr=boolean
  OFF4 : powerlib/Power Electronics/Ideal Switch  Ron=0.001  Lon=0  IC=0  Rs=1e5  Cs=inf  Measurements=off
      settings: SourceProductName=Simscape Electrical
  ON4 : powerlib/Power Electronics/Ideal Switch  Ron=0.001  Lon=0  IC=0  Rs=1e5  Cs=inf  Measurements=off
      settings: SourceProductName=Simscape Electrical
  Conn1 : PMIOPort  Side=Left
  Conn2 : PMIOPort  Port=2  Side=Right
  wires:
  Compare To Constat5/1 -> OFF4/1
  Clock7/1 -> Compare To Constat5/1, Compare To Constant4/1
  Compare To Constant4/1 -> ON4/1
  connections:
  ON4/RConn1 -- OFF4/LConn1
  OFF4/RConn1 -- Conn2/RConn1
  ON4/LConn1 -- Conn1/RConn1

== system Sim_Induct_Harmon/ON_OFF_18 ==
  Clock7 : Clock
  Compare To Constant4 : simulink/Logic and Bit Operations/Compare To Constant  relop=>=  const=sim_on(18)  OutDataTypeStr=boolean
  Compare To Constat5 : simulink/Logic and Bit Operations/Compare To Constant  relop=<=  const=sim_off(18)  OutDataTypeStr=boolean
  OFF4 : powerlib/Power Electronics/Ideal Switch  Ron=0.001  Lon=0  IC=0  Rs=1e5  Cs=inf  Measurements=off
      settings: SourceProductName=Simscape Electrical
  ON4 : powerlib/Power Electronics/Ideal Switch  Ron=0.001  Lon=0  IC=0  Rs=1e5  Cs=inf  Measurements=off
      settings: SourceProductName=Simscape Electrical
  Conn1 : PMIOPort  Side=Left
  Conn2 : PMIOPort  Port=2  Side=Right
  wires:
  Compare To Constat5/1 -> OFF4/1
  Clock7/1 -> Compare To Constat5/1, Compare To Constant4/1
  Compare To Constant4/1 -> ON4/1
  connections:
  ON4/RConn1 -- OFF4/LConn1
  OFF4/RConn1 -- Conn2/RConn1
  ON4/LConn1 -- Conn1/RConn1

== system Sim_Induct_Harmon/ON_OFF_19 ==
  Clock7 : Clock
  Compare To Constant4 : simulink/Logic and Bit Operations/Compare To Constant  relop=>=  const=sim_on(19)  OutDataTypeStr=boolean
  Compare To Constat5 : simulink/Logic and Bit Operations/Compare To Constant  relop=<=  const=sim_off(19)  OutDataTypeStr=boolean
  OFF4 : powerlib/Power Electronics/Ideal Switch  Ron=0.001  Lon=0  IC=0  Rs=1e5  Cs=inf  Measurements=off
      settings: SourceProductName=Simscape Electrical
  ON4 : powerlib/Power Electronics/Ideal Switch  Ron=0.001  Lon=0  IC=0  Rs=1e5  Cs=inf  Measurements=off
      settings: SourceProductName=Simscape Electrical
  Conn1 : PMIOPort  Side=Left
  Conn2 : PMIOPort  Port=2  Side=Right
  wires:
  Compare To Constat5/1 -> OFF4/1
  Clock7/1 -> Compare To Constat5/1, Compare To Constant4/1
  Compare To Constant4/1 -> ON4/1
  connections:
  ON4/RConn1 -- OFF4/LConn1
  OFF4/RConn1 -- Conn2/RConn1
  ON4/LConn1 -- Conn1/RConn1

== system Sim_Induct_Harmon/ON_OFF_2 ==
  Clock1 : Clock
  Clock2 : Clock
  Clock3 : Clock
  Compare To Constant : simulink/Logic and Bit Operations/Compare To Constant  relop=>=  const=sim_on(2)  OutDataTypeStr=boolean
  Compare To Constant1 : simulink/Logic and Bit Operations/Compare To Constant  relop=>=  const=sim_off(2)  OutDataTypeStr=boolean
  Compare To Constant2 : simulink/Logic and Bit Operations/Compare To Constant  relop=>=  const=sim_on(2)  OutDataTypeStr=boolean
  Constant : Constant  Value=0
  Constant1 : Constant  Value=0
  Ideal Switch : powerlib/Power Electronics/Ideal Switch  Ron=0.001  Lon=0  IC=0  Rs=1e5  Cs=inf  Measurements=off
      settings: SourceProductName=Simscape Electrical
  Switch : Switch
  Switch1 : Switch
  Conn1 : PMIOPort  Side=Left
  Conn2 : PMIOPort  Port=2  Side=Left
  tag scope: tensao_2=global
  wires:
  Switch1/1 -> [tensao_2]
  Constant/1 -> Switch/3
  Switch/1 -> Switch1/3
  Clock1/1 -> Compare To Constant/1
  Clock2/1 -> Compare To Constant1/1
  Compare To Constant1/1 -> Switch1/2
  [fonte_tensao] -> Switch/1
  Constant1/1 -> Switch1/1
  Compare To Constant/1 -> Switch/2
  Clock3/1 -> Compare To Constant2/1
  Compare To Constant2/1 -> Ideal Switch/1
  connections:
  Conn1/RConn1 -- Ideal Switch/LConn1
  Ideal Switch/RConn1 -- Conn2/RConn1

== system Sim_Induct_Harmon/ON_OFF_20 ==
  Clock7 : Clock
  Compare To Constant4 : simulink/Logic and Bit Operations/Compare To Constant  relop=>=  const=sim_on(20)  OutDataTypeStr=boolean
  Compare To Constat5 : simulink/Logic and Bit Operations/Compare To Constant  relop=<=  const=sim_off(20)  OutDataTypeStr=boolean
  OFF4 : powerlib/Power Electronics/Ideal Switch  Ron=0.001  Lon=0  IC=0  Rs=1e5  Cs=inf  Measurements=off
      settings: SourceProductName=Simscape Electrical
  ON4 : powerlib/Power Electronics/Ideal Switch  Ron=0.001  Lon=0  IC=0  Rs=1e5  Cs=inf  Measurements=off
      settings: SourceProductName=Simscape Electrical
  Conn1 : PMIOPort  Side=Left
  Conn2 : PMIOPort  Port=2  Side=Right
  wires:
  Compare To Constat5/1 -> OFF4/1
  Clock7/1 -> Compare To Constat5/1, Compare To Constant4/1
  Compare To Constant4/1 -> ON4/1
  connections:
  ON4/RConn1 -- OFF4/LConn1
  OFF4/RConn1 -- Conn2/RConn1
  ON4/LConn1 -- Conn1/RConn1

== system Sim_Induct_Harmon/ON_OFF_21 ==
  Clock8 : Clock
  Compare To Constant5 : simulink/Logic and Bit Operations/Compare To Constant  relop=>=  const=sim_on(21)  OutDataTypeStr=boolean
  Compare To Constat6 : simulink/Logic and Bit Operations/Compare To Constant  relop=<=  const=sim_off(21)  OutDataTypeStr=boolean
  OFF5 : powerlib/Power Electronics/Ideal Switch  Ron=0.001  Lon=0  IC=0  Rs=1e5  Cs=inf  Measurements=off
      settings: SourceProductName=Simscape Electrical
  ON5 : powerlib/Power Electronics/Ideal Switch  Ron=0.001  Lon=0  IC=0  Rs=1e5  Cs=inf  Measurements=off
      settings: SourceProductName=Simscape Electrical
  Conn1 : PMIOPort  Side=Left
  Conn2 : PMIOPort  Port=2  Side=Right
  wires:
  Clock8/1 -> Compare To Constat6/1, Compare To Constant5/1
  Compare To Constat6/1 -> OFF5/1
  Compare To Constant5/1 -> ON5/1
  connections:
  ON5/RConn1 -- OFF5/LConn1
  OFF5/RConn1 -- Conn2/RConn1
  ON5/LConn1 -- Conn1/RConn1

== system Sim_Induct_Harmon/ON_OFF_22 ==
  Clock8 : Clock
  Compare To Constant5 : simulink/Logic and Bit Operations/Compare To Constant  relop=>=  const=sim_on(22)  OutDataTypeStr=boolean
  Compare To Constat6 : simulink/Logic and Bit Operations/Compare To Constant  relop=<=  const=sim_off(22)  OutDataTypeStr=boolean
  OFF5 : powerlib/Power Electronics/Ideal Switch  Ron=0.001  Lon=0  IC=0  Rs=1e5  Cs=inf  Measurements=off
      settings: SourceProductName=Simscape Electrical
  ON5 : powerlib/Power Electronics/Ideal Switch  Ron=0.001  Lon=0  IC=0  Rs=1e5  Cs=inf  Measurements=off
      settings: SourceProductName=Simscape Electrical
  Conn1 : PMIOPort  Side=Left
  Conn2 : PMIOPort  Port=2  Side=Right
  wires:
  Clock8/1 -> Compare To Constat6/1, Compare To Constant5/1
  Compare To Constat6/1 -> OFF5/1
  Compare To Constant5/1 -> ON5/1
  connections:
  ON5/RConn1 -- OFF5/LConn1
  OFF5/RConn1 -- Conn2/RConn1
  ON5/LConn1 -- Conn1/RConn1

== system Sim_Induct_Harmon/ON_OFF_23 ==
  Clock8 : Clock
  Compare To Constant5 : simulink/Logic and Bit Operations/Compare To Constant  relop=>=  const=sim_on(23)  OutDataTypeStr=boolean
  Compare To Constat6 : simulink/Logic and Bit Operations/Compare To Constant  relop=<=  const=sim_off(23)  OutDataTypeStr=boolean
  OFF5 : powerlib/Power Electronics/Ideal Switch  Ron=0.001  Lon=0  IC=0  Rs=1e5  Cs=inf  Measurements=off
      settings: SourceProductName=Simscape Electrical
  ON5 : powerlib/Power Electronics/Ideal Switch  Ron=0.001  Lon=0  IC=0  Rs=1e5  Cs=inf  Measurements=off
      settings: SourceProductName=Simscape Electrical
  Conn1 : PMIOPort  Side=Left
  Conn2 : PMIOPort  Port=2  Side=Right
  wires:
  Clock8/1 -> Compare To Constat6/1, Compare To Constant5/1
  Compare To Constat6/1 -> OFF5/1
  Compare To Constant5/1 -> ON5/1
  connections:
  ON5/RConn1 -- OFF5/LConn1
  OFF5/RConn1 -- Conn2/RConn1
  ON5/LConn1 -- Conn1/RConn1

== system Sim_Induct_Harmon/ON_OFF_24 ==
  Clock8 : Clock
  Compare To Constant5 : simulink/Logic and Bit Operations/Compare To Constant  relop=>=  const=sim_on(24)  OutDataTypeStr=boolean
  Compare To Constat6 : simulink/Logic and Bit Operations/Compare To Constant  relop=<=  const=sim_off(24)  OutDataTypeStr=boolean
  OFF5 : powerlib/Power Electronics/Ideal Switch  Ron=0.001  Lon=0  IC=0  Rs=1e5  Cs=inf  Measurements=off
      settings: SourceProductName=Simscape Electrical
  ON5 : powerlib/Power Electronics/Ideal Switch  Ron=0.001  Lon=0  IC=0  Rs=1e5  Cs=inf  Measurements=off
      settings: SourceProductName=Simscape Electrical
  Conn1 : PMIOPort  Side=Left
  Conn2 : PMIOPort  Port=2  Side=Right
  wires:
  Clock8/1 -> Compare To Constat6/1, Compare To Constant5/1
  Compare To Constat6/1 -> OFF5/1
  Compare To Constant5/1 -> ON5/1
  connections:
  ON5/RConn1 -- OFF5/LConn1
  OFF5/RConn1 -- Conn2/RConn1
  ON5/LConn1 -- Conn1/RConn1

== system Sim_Induct_Harmon/ON_OFF_25 ==
  Clock8 : Clock
  Compare To Constant5 : simulink/Logic and Bit Operations/Compare To Constant  relop=>=  const=sim_on(25)  OutDataTypeStr=boolean
  Compare To Constat6 : simulink/Logic and Bit Operations/Compare To Constant  relop=<=  const=sim_off(25)  OutDataTypeStr=boolean
  OFF5 : powerlib/Power Electronics/Ideal Switch  Ron=0.001  Lon=0  IC=0  Rs=1e5  Cs=inf  Measurements=off
      settings: SourceProductName=Simscape Electrical
  ON5 : powerlib/Power Electronics/Ideal Switch  Ron=0.001  Lon=0  IC=0  Rs=1e5  Cs=inf  Measurements=off
      settings: SourceProductName=Simscape Electrical
  Conn1 : PMIOPort  Side=Left
  Conn2 : PMIOPort  Port=2  Side=Right
  wires:
  Clock8/1 -> Compare To Constat6/1, Compare To Constant5/1
  Compare To Constat6/1 -> OFF5/1
  Compare To Constant5/1 -> ON5/1
  connections:
  ON5/RConn1 -- OFF5/LConn1
  OFF5/RConn1 -- Conn2/RConn1
  ON5/LConn1 -- Conn1/RConn1
